simulink model "OOCconSoloEspEst"  (R2020a)
settings: Solver=VariableStepAuto  StartTime=0.0  StopTime=1000  RelTol=1e-3
settings Model: Creator=Sergio  LastModifiedBy=Sergio

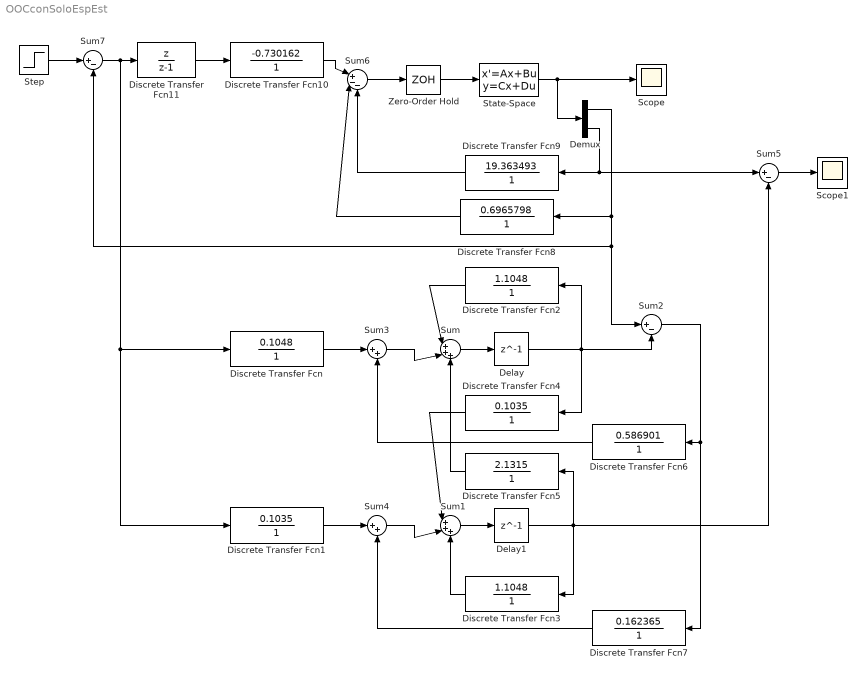
== system OOCconSoloEspEst ==
  Delay : Delay  DelayLength=1
  Delay1 : Delay  DelayLength=1
  Demux : Demux  Outputs=2
  Discrete Transfer Fcn : DiscreteTransferFcn  Numerator=[0.1048]  Denominator=[1]
  Discrete Transfer Fcn1 : DiscreteTransferFcn  Numerator=[0.1035]  Denominator=[1]
  Discrete Transfer Fcn10 : DiscreteTransferFcn  Numerator=[-0.730162]  Denominator=[1]
  Discrete Transfer Fcn11 : DiscreteTransferFcn  Numerator=[1 0]  Denominator=[1 -1]
  Discrete Transfer Fcn2 : DiscreteTransferFcn  Numerator=[1.1048]  Denominator=[1]
  Discrete Transfer Fcn3 : DiscreteTransferFcn  Numerator=[1.1048]  Denominator=[1]
  Discrete Transfer Fcn4 : DiscreteTransferFcn  Numerator=[0.1035]  Denominator=[1]
  Discrete Transfer Fcn5 : DiscreteTransferFcn  Numerator=[2.1315]  Denominator=[1]
  Discrete Transfer Fcn6 : DiscreteTransferFcn  Numerator=[0.586901]  Denominator=[1]
  Discrete Transfer Fcn7 : DiscreteTransferFcn  Numerator=[0.162365]  Denominator=[1]
  Discrete Transfer Fcn8 : DiscreteTransferFcn  Numerator=[0.6965798]  Denominator=[1]
  Discrete Transfer Fcn9 : DiscreteTransferFcn  Numerator=[19.363493]  Denominator=[1]
  Scope : Scope
  Scope1 : Scope
  State-Space : StateSpace  A=[0 20.6; 1 0]  B=[0; 1]  C=[1 0; 0 1]  D=[0; 0]  InitialCondition=[1; 0]
  Step : Step  SampleTime=0
  Sum : Sum  Inputs=|+++
  Sum1 : Sum  Inputs=|+++
  Sum2 : Sum  Inputs=|+-
  Sum3 : Sum  Inputs=|++
  Sum4 : Sum  Inputs=|++
  Sum5 : Sum  Inputs=|+-
  Sum6 : Sum  Inputs=|+--
  Sum7 : Sum  Inputs=|+-
  Zero-Order Hold : ZeroOrderHold  SampleTime=0.1
  wires:
  State-Space/1 -> Demux/1, Scope/1
  Zero-Order Hold/1 -> State-Space/1
  Sum/1 -> Delay/1
  Sum1/1 -> Delay1/1
  Discrete Transfer Fcn/1 -> Sum3/1
  Discrete Transfer Fcn1/1 -> Sum4/1
  Delay/1 -> Discrete Transfer Fcn4/1, Discrete Transfer Fcn2/1, Sum2/2
  Sum3/1 -> Sum/2
  Sum4/1 -> Sum1/2
  Discrete Transfer Fcn2/1 -> Sum/1
  Delay1/1 -> Sum5/2, Discrete Transfer Fcn5/1, Discrete Transfer Fcn3/1
  Discrete Transfer Fcn3/1 -> Sum1/3
  Discrete Transfer Fcn4/1 -> Sum1/1
  Discrete Transfer Fcn5/1 -> Sum/3
  Sum2/1 -> Discrete Transfer Fcn7/1, Discrete Transfer Fcn6/1
  Discrete Transfer Fcn6/1 -> Sum3/2
  Discrete Transfer Fcn7/1 -> Sum4/2
  Sum5/1 -> Scope1/1
  Sum6/1 -> Zero-Order Hold/1
  Demux/1 -> Sum7/2, Sum2/1, Discrete Transfer Fcn8/1
  Demux/2 -> Sum5/1, Discrete Transfer Fcn9/1
  Discrete Transfer Fcn9/1 -> Sum6/3
  Discrete Transfer Fcn8/1 -> Sum6/2
  Discrete Transfer Fcn10/1 -> Sum6/1
  Discrete Transfer Fcn11/1 -> Discrete Transfer Fcn10/1
  Sum7/1 -> Discrete Transfer Fcn1/1, Discrete Transfer Fcn/1, Discrete Transfer Fcn11/1
  Step/1 -> Sum7/1
